simulink model "NDT_Localization"  (R2022a)
settings: Solver=FixedStepAuto  StartTime=0.0  StopTime=10.0  RelTol=1e-3
model workspace (MAT data in the model file):
  SL_ROS_VariableLengthArrays_MaxSizes : object (value not decoded)
undefined symbols (not defined in the file or in its folder): null
libraries: ros2lib x9, robotlib x8, simulink x1
(part 10 of 12)

== system NDT_Localization/observation_callback/check_localizer/If Action Subsystem/register_measurement_impl/If Action Subsystem/If Action Subsystem/solve/If Action Subsystem1/For Iterator Subsystem/compute_next_step/If Action Subsystem1/For Iterator Subsystem/If Action Subsystem/If Action Subsystem3/If Action Subsystem/f_u/For Iterator Subsystem/score ==
  score : Inport
  sigma : Inport  Port=2
  myu : Inport  Port=3
  x : Inport  Port=4
  d1 : Inport  Port=5
  d2 : Inport  Port=6
  Add : Sum  Inputs=+-
  Add1 : Sum
  Constant : Constant  Value=-2
  Divide1 : Product  Inputs=*/
  Gain : Gain  Gain=-1
  Math Function : Math
  Math Function1 : Math  Operator=transpose
  Math Function2 : Math  Operator=reciprocal
  Product : Product
  Product1 : Product  Inputs=3  Multiplication=Matrix(*)
  Product2 : Product
  p : Outport
  wires:
  sigma/1 -> Math Function2/1
  Math Function/1 -> Product/2
  Gain/1 -> Product/1  "-d1"
  myu/1 -> Add/2
  x/1 -> Add/1
  Product2/1 -> Math Function/1
  Add/1 -> Product1/3, Math Function1/1  "x-myu"
  Product/1 -> Add1/2
  Math Function1/1 -> Product1/1
  Product1/1 -> Product2/2
  Math Function2/1 -> Product1/2
  Constant/1 -> Divide1/2
  Divide1/1 -> Product2/1
  d2/1 -> Divide1/1  "d2"
  d1/1 -> Gain/1
  Add1/1 -> p/1
  score/1 -> Add1/1

== system NDT_Localization/observation_callback/check_localizer/If Action Subsystem/register_measurement_impl/If Action Subsystem/If Action Subsystem/solve/If Action Subsystem1/For Iterator Subsystem/compute_next_step/If Action Subsystem1/For Iterator Subsystem/If Action Subsystem/If Action Subsystem3/If Action Subsystem/f_u/angle_params/If Action Subsystem ==
  Action Port : ActionPort
  Constant : Constant
  Constant1 : Constant  Value=0
  Out1 : Outport
  Out2 : Outport  Port=2
  wires:
  Constant/1 -> Out1/1
  Constant1/1 -> Out2/1

== system NDT_Localization/observation_callback/check_localizer/If Action Subsystem/register_measurement_impl/If Action Subsystem/If Action Subsystem/solve/If Action Subsystem1/For Iterator Subsystem/compute_next_step/If Action Subsystem1/For Iterator Subsystem/If Action Subsystem/If Action Subsystem3/If Action Subsystem/f_u/angle_params/If Action Subsystem1 ==
  x : Inport
  Action Port : ActionPort
  Trigonometric Function : Trigonometry  Operator=cos
  Trigonometric Function1 : Trigonometry
  Out1 : Outport
  Out2 : Outport  Port=2
  wires:
  x/1 -> Trigonometric Function1/1, Trigonometric Function/1
  Trigonometric Function1/1 -> Out2/1
  Trigonometric Function/1 -> Out1/1

== system NDT_Localization/observation_callback/check_localizer/If Action Subsystem/register_measurement_impl/If Action Subsystem/If Action Subsystem/solve/If Action Subsystem1/For Iterator Subsystem/compute_next_step/If Action Subsystem1/For Iterator Subsystem/If Action Subsystem/If Action Subsystem3/If Action Subsystem/f_u/angle_params/If Action Subsystem2 ==
  Action Port : ActionPort
  Constant : Constant
  Constant1 : Constant  Value=0
  Out1 : Outport
  Out2 : Outport  Port=2
  wires:
  Constant/1 -> Out1/1
  Constant1/1 -> Out2/1

== system NDT_Localization/observation_callback/check_localizer/If Action Subsystem/register_measurement_impl/If Action Subsystem/If Action Subsystem/solve/If Action Subsystem1/For Iterator Subsystem/compute_next_step/If Action Subsystem1/For Iterator Subsystem/If Action Subsystem/If Action Subsystem3/If Action Subsystem/f_u/angle_params/If Action Subsystem3 ==
  y : Inport
  Action Port : ActionPort
  Trigonometric Function : Trigonometry  Operator=cos
  Trigonometric Function1 : Trigonometry
  Out1 : Outport
  Out2 : Outport  Port=2
  wires:
  Trigonometric Function/1 -> Out1/1
  Trigonometric Function1/1 -> Out2/1
  y/1 -> Trigonometric Function1/1, Trigonometric Function/1

== system NDT_Localization/observation_callback/check_localizer/If Action Subsystem/register_measurement_impl/If Action Subsystem/If Action Subsystem/solve/If Action Subsystem1/For Iterator Subsystem/compute_next_step/If Action Subsystem1/For Iterator Subsystem/If Action Subsystem/If Action Subsystem3/If Action Subsystem/f_u/angle_params/If Action Subsystem4 ==
  Action Port : ActionPort
  Constant : Constant
  Constant1 : Constant  Value=0
  Out1 : Outport
  Out2 : Outport  Port=2
  wires:
  Constant/1 -> Out1/1
  Constant1/1 -> Out2/1

== system NDT_Localization/observation_callback/check_localizer/If Action Subsystem/register_measurement_impl/If Action Subsystem/If Action Subsystem/solve/If Action Subsystem1/For Iterator Subsystem/compute_next_step/If Action Subsystem1/For Iterator Subsystem/If Action Subsystem/If Action Subsystem3/If Action Subsystem/f_u/angle_params/If Action Subsystem5 ==
  z : Inport
  Action Port : ActionPort
  Trigonometric Function : Trigonometry  Operator=cos
  Trigonometric Function1 : Trigonometry
  Out1 : Outport
  Out2 : Outport  Port=2
  wires:
  Trigonometric Function1/1 -> Out2/1
  Trigonometric Function/1 -> Out1/1
  z/1 -> Trigonometric Function1/1, Trigonometric Function/1

== system NDT_Localization/observation_callback/check_localizer/If Action Subsystem/register_measurement_impl/If Action Subsystem/If Action Subsystem/solve/If Action Subsystem1/For Iterator Subsystem/compute_next_step/If Action Subsystem1/For Iterator Subsystem/If Action Subsystem/If Action Subsystem3/psi_t/initial_objective_function/For Iterator Subsystem/gradient_jaco ==
  set_jacobian : Inport
  set_gradient : Inport  Port=2
  index : Inport  Port=3
  data : Inport  Port=4
  sigma : Inport  Port=5
  myu : Inport  Port=6
  x : Inport  Port=7
  d1 : Inport  Port=8
  d2 : Inport  Port=9
  Add : Sum  Inputs=+-
  Constant : Constant  Value=-2
  Divide1 : Product  Inputs=*/
  Math Function : Math
  Math Function1 : Math  Operator=transpose
  Math Function2 : Math  Operator=reciprocal
  Product : Product  Inputs=4
  Product1 : Product  Inputs=3  Multiplication=Matrix(*)
  Product2 : Product
  Product3 : Product
  Product4 : Product  Multiplication=Matrix(*)
  gradient_col : MATLAB Function  TreatAsAtomicUnit=on
  jaco_add : MATLAB Function  TreatAsAtomicUnit=on
  Out1 : Outport
  wires:
  myu/1 -> Add/2
  Constant/1 -> Divide1/2
  Math Function1/1 -> Product1/1
  Divide1/1 -> Product2/1
  d2/1 -> Divide1/1, Product/3  "d2"
  Math Function2/1 -> Product3/2, Product1/2  "inv_cov"
  Product1/1 -> Product2/2
  d1/1 -> Product/2  "d1"
  x/1 -> Add/1
  Math Function/1 -> Product/4
  Product2/1 -> Math Function/1
  Add/1 -> Product1/3, Math Function1/1  "x-myu"
  sigma/1 -> Math Function2/1
  Product/1 -> jaco_add/3(num)
  index/1 -> jaco_add/2(index), gradient_col/1(index)
  jaco_add/1(jacobian) -> Out1/1
  set_jacobian/1 -> jaco_add/1("jacobian ")
  set_gradient/1 -> gradient_col/2(gradient)
  gradient_col/1(y) -> Product3/1
  data/1 -> Product4/1
  Product3/1 -> Product4/2
  Product4/1 -> Product/1

== system NDT_Localization/observation_callback/check_localizer/If Action Subsystem/register_measurement_impl/If Action Subsystem/If Action Subsystem/solve/If Action Subsystem1/For Iterator Subsystem/compute_next_step/If Action Subsystem1/For Iterator Subsystem/If Action Subsystem/If Action Subsystem3/psi_t/initial_objective_function/For Iterator Subsystem/make_c_param ==
  outlier_ratio : Inport
  voxel_size_x : Inport  Port=2
  voxel_size_y : Inport  Port=3
  voxel_size_z : Inport  Port=4
  Constant : Constant
  Divide : Product  Inputs=*/
  Gain : Gain  Gain=10
  Product : Product  Inputs=3
  Subtract : Sum  Inputs=+-
  c1 : Outport
  c2 : Outport  Port=2
  wires:
  Constant/1 -> Subtract/1
  outlier_ratio/1 -> Divide/1, Subtract/2
  Subtract/1 -> Gain/1
  Gain/1 -> c1/1
  Product/1 -> Divide/2
  Divide/1 -> c2/1
  voxel_size_y/1 -> Product/2
  voxel_size_z/1 -> Product/3
  voxel_size_x/1 -> Product/1

== system NDT_Localization/observation_callback/check_localizer/If Action Subsystem/register_measurement_impl/If Action Subsystem/If Action Subsystem/solve/If Action Subsystem1/For Iterator Subsystem/compute_next_step/If Action Subsystem1/For Iterator Subsystem/If Action Subsystem/If Action Subsystem3/psi_t/initial_objective_function/For Iterator Subsystem/make_d_param ==
  c1 : Inport
  c2 : Inport  Port=2
  Add1 : Sum
  Add2 : Sum  Inputs=-+
  Add3 : Sum
  Add4 : Sum  Inputs=+-
  Constant : Constant  Value=-2
  Constant1 : Constant  Value=-0.5
  Divide : Product  Inputs=*/
  Math Function{3..4,6..7} (4 alike) : Math  Operator=log
  Math Function5 : Math
  Product3 : Product
  Product4 : Product
  d1 : Outport
  d2 : Outport  Port=2
  wires:
  Add2/1 -> Divide/2, d1/1  "d1"
  Math Function4/1 -> Add4/1, Add2/2  "-d3"
  Product4/1 -> Add3/1
  Add3/1 -> Math Function6/1
  c1/1 -> Product4/1, Add1/1
  Constant/1 -> Product3/2
  Constant1/1 -> Math Function5/1
  Product3/1 -> d2/1  "d2"
  Math Function5/1 -> Product4/2
  Math Function7/1 -> Product3/1
  Divide/1 -> Math Function7/1
  Math Function6/1 -> Add4/2
  c2/1 -> Add3/2, Math Function4/1, Add1/2
  Add4/1 -> Divide/1
  Add1/1 -> Math Function3/1
  Math Function3/1 -> Add2/1

== system NDT_Localization/observation_callback/check_localizer/If Action Subsystem/register_measurement_impl/If Action Subsystem/If Action Subsystem/solve/If Action Subsystem1/For Iterator Subsystem/compute_next_step/If Action Subsystem1/For Iterator Subsystem/If Action Subsystem/If Action Subsystem3/psi_t/initial_objective_function/For Iterator Subsystem/score ==
  score : Inport
  sigma : Inport  Port=2
  myu : Inport  Port=3
  x : Inport  Port=4
  d1 : Inport  Port=5
  d2 : Inport  Port=6
  Add : Sum  Inputs=+-
  Add1 : Sum
  Constant : Constant  Value=-2
  Divide1 : Product  Inputs=*/
  Gain : Gain  Gain=-1
  Math Function : Math
  Math Function1 : Math  Operator=transpose
  Math Function2 : Math  Operator=reciprocal
  Product : Product
  Product1 : Product  Inputs=3  Multiplication=Matrix(*)
  Product2 : Product
  p : Outport
  wires:
  sigma/1 -> Math Function2/1
  Math Function/1 -> Product/2
  Gain/1 -> Product/1  "-d1"
  myu/1 -> Add/2
  x/1 -> Add/1
  Product2/1 -> Math Function/1
  Add/1 -> Product1/3, Math Function1/1  "x-myu"
  Product/1 -> Add1/2
  Math Function1/1 -> Product1/1
  Product1/1 -> Product2/2
  Math Function2/1 -> Product1/2
  Constant/1 -> Divide1/2
  Divide1/1 -> Product2/1
  d2/1 -> Divide1/1  "d2"
  d1/1 -> Gain/1
  Add1/1 -> p/1
  score/1 -> Add1/1

== system NDT_Localization/observation_callback/check_localizer/If Action Subsystem/register_measurement_impl/If Action Subsystem/If Action Subsystem/solve/If Action Subsystem1/For Iterator Subsystem/compute_next_step/If Action Subsystem1/For Iterator Subsystem/If Action Subsystem/If Action Subsystem3/psi_t/initial_objective_function/angle_params/If Action Subsystem ==
  Action Port : ActionPort
  Constant : Constant
  Constant1 : Constant  Value=0
  Out1 : Outport
  Out2 : Outport  Port=2
  wires:
  Constant/1 -> Out1/1
  Constant1/1 -> Out2/1

== system NDT_Localization/observation_callback/check_localizer/If Action Subsystem/register_measurement_impl/If Action Subsystem/If Action Subsystem/solve/If Action Subsystem1/For Iterator Subsystem/compute_next_step/If Action Subsystem1/For Iterator Subsystem/If Action Subsystem/If Action Subsystem3/psi_t/initial_objective_function/angle_params/If Action Subsystem1 ==
  x : Inport
  Action Port : ActionPort
  Trigonometric Function : Trigonometry  Operator=cos
  Trigonometric Function1 : Trigonometry
  Out1 : Outport
  Out2 : Outport  Port=2
  wires:
  x/1 -> Trigonometric Function1/1, Trigonometric Function/1
  Trigonometric Function1/1 -> Out2/1
  Trigonometric Function/1 -> Out1/1

== system NDT_Localization/observation_callback/check_localizer/If Action Subsystem/register_measurement_impl/If Action Subsystem/If Action Subsystem/solve/If Action Subsystem1/For Iterator Subsystem/compute_next_step/If Action Subsystem1/For Iterator Subsystem/If Action Subsystem/If Action Subsystem3/psi_t/initial_objective_function/angle_params/If Action Subsystem2 ==
  Action Port : ActionPort
  Constant : Constant
  Constant1 : Constant  Value=0
  Out1 : Outport
  Out2 : Outport  Port=2
  wires:
  Constant/1 -> Out1/1
  Constant1/1 -> Out2/1

== system NDT_Localization/observation_callback/check_localizer/If Action Subsystem/register_measurement_impl/If Action Subsystem/If Action Subsystem/solve/If Action Subsystem1/For Iterator Subsystem/compute_next_step/If Action Subsystem1/For Iterator Subsystem/If Action Subsystem/If Action Subsystem3/psi_t/initial_objective_function/angle_params/If Action Subsystem3 ==
  y : Inport
  Action Port : ActionPort
  Trigonometric Function : Trigonometry  Operator=cos
  Trigonometric Function1 : Trigonometry
  Out1 : Outport
  Out2 : Outport  Port=2
  wires:
  Trigonometric Function/1 -> Out1/1
  Trigonometric Function1/1 -> Out2/1
  y/1 -> Trigonometric Function1/1, Trigonometric Function/1

== system NDT_Localization/observation_callback/check_localizer/If Action Subsystem/register_measurement_impl/If Action Subsystem/If Action Subsystem/solve/If Action Subsystem1/For Iterator Subsystem/compute_next_step/If Action Subsystem1/For Iterator Subsystem/If Action Subsystem/If Action Subsystem3/psi_t/initial_objective_function/angle_params/If Action Subsystem4 ==
  Action Port : ActionPort
  Constant : Constant
  Constant1 : Constant  Value=0
  Out1 : Outport
  Out2 : Outport  Port=2
  wires:
  Constant/1 -> Out1/1
  Constant1/1 -> Out2/1

== system NDT_Localization/observation_callback/check_localizer/If Action Subsystem/register_measurement_impl/If Action Subsystem/If Action Subsystem/solve/If Action Subsystem1/For Iterator Subsystem/compute_next_step/If Action Subsystem1/For Iterator Subsystem/If Action Subsystem/If Action Subsystem3/psi_t/initial_objective_function/angle_params/If Action Subsystem5 ==
  z : Inport
  Action Port : ActionPort
  Trigonometric Function : Trigonometry  Operator=cos
  Trigonometric Function1 : Trigonometry
  Out1 : Outport
  Out2 : Outport  Port=2
  wires:
  Trigonometric Function1/1 -> Out2/1
  Trigonometric Function/1 -> Out1/1
  z/1 -> Trigonometric Function1/1, Trigonometric Function/1

== system NDT_Localization/observation_callback/check_localizer/If Action Subsystem/register_measurement_impl/If Action Subsystem/If Action Subsystem/solve/If Action Subsystem1/For Iterator Subsystem/compute_next_step/If Action Subsystem1/For Iterator Subsystem/If Action Subsystem/If Action Subsystem3/psi_t/objective_function/For Iterator Subsystem/gradient_jaco ==
  set_jacobian : Inport
  set_gradient : Inport  Port=2
  index : Inport  Port=3
  data : Inport  Port=4
  sigma : Inport  Port=5
  myu : Inport  Port=6
  x : Inport  Port=7
  d1 : Inport  Port=8
  d2 : Inport  Port=9
  Add : Sum  Inputs=+-
  Constant : Constant  Value=-2
  Divide1 : Product  Inputs=*/
  Math Function : Math
  Math Function1 : Math  Operator=transpose
  Math Function2 : Math  Operator=reciprocal
  Product : Product  Inputs=4
  Product1 : Product  Inputs=3  Multiplication=Matrix(*)
  Product2 : Product
  Product3 : Product
  Product4 : Product  Multiplication=Matrix(*)
  gradient_col : MATLAB Function  TreatAsAtomicUnit=on
  jaco_add : MATLAB Function  TreatAsAtomicUnit=on
  Out1 : Outport
  wires:
  myu/1 -> Add/2
  Constant/1 -> Divide1/2
  Math Function1/1 -> Product1/1
  Divide1/1 -> Product2/1
  d2/1 -> Divide1/1, Product/3  "d2"
  Math Function2/1 -> Product3/2, Product1/2  "inv_cov"
  Product1/1 -> Product2/2
  d1/1 -> Product/2  "d1"
  x/1 -> Add/1
  Math Function/1 -> Product/4
  Product2/1 -> Math Function/1
  Add/1 -> Product1/3, Math Function1/1  "x-myu"
  sigma/1 -> Math Function2/1
  Product/1 -> jaco_add/3(num)
  index/1 -> jaco_add/2(index), gradient_col/1(index)
  jaco_add/1(jacobian) -> Out1/1
  set_jacobian/1 -> jaco_add/1("jacobian ")
  set_gradient/1 -> gradient_col/2(gradient)
  gradient_col/1(y) -> Product3/1
  data/1 -> Product4/1
  Product3/1 -> Product4/2
  Product4/1 -> Product/1

== system NDT_Localization/observation_callback/check_localizer/If Action Subsystem/register_measurement_impl/If Action Subsystem/If Action Subsystem/solve/If Action Subsystem1/For Iterator Subsystem/compute_next_step/If Action Subsystem1/For Iterator Subsystem/If Action Subsystem/If Action Subsystem3/psi_t/objective_function/For Iterator Subsystem/make_c_param ==
  outlier_ratio : Inport
  voxel_size_x : Inport  Port=2
  voxel_size_y : Inport  Port=3
  voxel_size_z : Inport  Port=4
  Constant : Constant
  Divide : Product  Inputs=*/
  Gain : Gain  Gain=10
  Product : Product  Inputs=3
  Subtract : Sum  Inputs=+-
  c1 : Outport
  c2 : Outport  Port=2
  wires:
  Constant/1 -> Subtract/1
  outlier_ratio/1 -> Divide/1, Subtract/2
  Subtract/1 -> Gain/1
  Gain/1 -> c1/1
  Product/1 -> Divide/2
  Divide/1 -> c2/1
  voxel_size_y/1 -> Product/2
  voxel_size_z/1 -> Product/3
  voxel_size_x/1 -> Product/1

== system NDT_Localization/observation_callback/check_localizer/If Action Subsystem/register_measurement_impl/If Action Subsystem/If Action Subsystem/solve/If Action Subsystem1/For Iterator Subsystem/compute_next_step/If Action Subsystem1/For Iterator Subsystem/If Action Subsystem/If Action Subsystem3/psi_t/objective_function/For Iterator Subsystem/make_d_param ==
  c1 : Inport
  c2 : Inport  Port=2
  Add1 : Sum
  Add2 : Sum  Inputs=-+
  Add3 : Sum
  Add4 : Sum  Inputs=+-
  Constant : Constant  Value=-2
  Constant1 : Constant  Value=-0.5
  Divide : Product  Inputs=*/
  Math Function{3..4,6..7} (4 alike) : Math  Operator=log
  Math Function5 : Math
  Product3 : Product
  Product4 : Product
  d1 : Outport
  d2 : Outport  Port=2
  wires:
  Add2/1 -> Divide/2, d1/1  "d1"
  Math Function4/1 -> Add4/1, Add2/2  "-d3"
  Product4/1 -> Add3/1
  Add3/1 -> Math Function6/1
  c1/1 -> Product4/1, Add1/1
  Constant/1 -> Product3/2
  Constant1/1 -> Math Function5/1
  Product3/1 -> d2/1  "d2"
  Math Function5/1 -> Product4/2
  Math Function7/1 -> Product3/1
  Divide/1 -> Math Function7/1
  Math Function6/1 -> Add4/2
  c2/1 -> Add3/2, Math Function4/1, Add1/2
  Add4/1 -> Divide/1
  Add1/1 -> Math Function3/1
  Math Function3/1 -> Add2/1

== system NDT_Localization/observation_callback/check_localizer/If Action Subsystem/register_measurement_impl/If Action Subsystem/If Action Subsystem/solve/If Action Subsystem1/For Iterator Subsystem/compute_next_step/If Action Subsystem1/For Iterator Subsystem/If Action Subsystem/If Action Subsystem3/psi_t/objective_function/For Iterator Subsystem/score ==
  score : Inport
  sigma : Inport  Port=2
  myu : Inport  Port=3
  x : Inport  Port=4
  d1 : Inport  Port=5
  d2 : Inport  Port=6
  Add : Sum  Inputs=+-
  Add1 : Sum
  Constant : Constant  Value=-2
  Divide1 : Product  Inputs=*/
  Gain : Gain  Gain=-1
  Math Function : Math
  Math Function1 : Math  Operator=transpose
  Math Function2 : Math  Operator=reciprocal
  Product : Product
  Product1 : Product  Inputs=3  Multiplication=Matrix(*)
  Product2 : Product
  p : Outport
  wires:
  sigma/1 -> Math Function2/1
  Math Function/1 -> Product/2
  Gain/1 -> Product/1  "-d1"
  myu/1 -> Add/2
  x/1 -> Add/1
  Product2/1 -> Math Function/1
  Add/1 -> Product1/3, Math Function1/1  "x-myu"
  Product/1 -> Add1/2
  Math Function1/1 -> Product1/1
  Product1/1 -> Product2/2
  Math Function2/1 -> Product1/2
  Constant/1 -> Divide1/2
  Divide1/1 -> Product2/1
  d2/1 -> Divide1/1  "d2"
  d1/1 -> Gain/1
  Add1/1 -> p/1
  score/1 -> Add1/1

== system NDT_Localization/observation_callback/check_localizer/If Action Subsystem/register_measurement_impl/If Action Subsystem/If Action Subsystem/solve/If Action Subsystem1/For Iterator Subsystem/compute_next_step/If Action Subsystem1/For Iterator Subsystem/If Action Subsystem/If Action Subsystem3/psi_t/objective_function/angle_params/If Action Subsystem ==
  Action Port : ActionPort
  Constant : Constant
  Constant1 : Constant  Value=0
  Out1 : Outport
  Out2 : Outport  Port=2
  wires:
  Constant/1 -> Out1/1
  Constant1/1 -> Out2/1

== system NDT_Localization/observation_callback/check_localizer/If Action Subsystem/register_measurement_impl/If Action Subsystem/If Action Subsystem/solve/If Action Subsystem1/For Iterator Subsystem/compute_next_step/If Action Subsystem1/For Iterator Subsystem/If Action Subsystem/If Action Subsystem3/psi_t/objective_function/angle_params/If Action Subsystem1 ==
  x : Inport
  Action Port : ActionPort
  Trigonometric Function : Trigonometry  Operator=cos
  Trigonometric Function1 : Trigonometry
  Out1 : Outport
  Out2 : Outport  Port=2
  wires:
  x/1 -> Trigonometric Function1/1, Trigonometric Function/1
  Trigonometric Function1/1 -> Out2/1
  Trigonometric Function/1 -> Out1/1

== system NDT_Localization/observation_callback/check_localizer/If Action Subsystem/register_measurement_impl/If Action Subsystem/If Action Subsystem/solve/If Action Subsystem1/For Iterator Subsystem/compute_next_step/If Action Subsystem1/For Iterator Subsystem/If Action Subsystem/If Action Subsystem3/psi_t/objective_function/angle_params/If Action Subsystem2 ==
  Action Port : ActionPort
  Constant : Constant
  Constant1 : Constant  Value=0
  Out1 : Outport
  Out2 : Outport  Port=2
  wires:
  Constant/1 -> Out1/1
  Constant1/1 -> Out2/1

== system NDT_Localization/observation_callback/check_localizer/If Action Subsystem/register_measurement_impl/If Action Subsystem/If Action Subsystem/solve/If Action Subsystem1/For Iterator Subsystem/compute_next_step/If Action Subsystem1/For Iterator Subsystem/If Action Subsystem/If Action Subsystem3/psi_t/objective_function/angle_params/If Action Subsystem3 ==
  y : Inport
  Action Port : ActionPort
  Trigonometric Function : Trigonometry  Operator=cos
  Trigonometric Function1 : Trigonometry
  Out1 : Outport
  Out2 : Outport  Port=2
  wires:
  Trigonometric Function/1 -> Out1/1
  Trigonometric Function1/1 -> Out2/1
  y/1 -> Trigonometric Function1/1, Trigonometric Function/1

== system NDT_Localization/observation_callback/check_localizer/If Action Subsystem/register_measurement_impl/If Action Subsystem/If Action Subsystem/solve/If Action Subsystem1/For Iterator Subsystem/compute_next_step/If Action Subsystem1/For Iterator Subsystem/If Action Subsystem/If Action Subsystem3/psi_t/objective_function/angle_params/If Action Subsystem4 ==
  Action Port : ActionPort
  Constant : Constant
  Constant1 : Constant  Value=0
  Out1 : Outport
  Out2 : Outport  Port=2
  wires:
  Constant/1 -> Out1/1
  Constant1/1 -> Out2/1

== system NDT_Localization/observation_callback/check_localizer/If Action Subsystem/register_measurement_impl/If Action Subsystem/If Action Subsystem/solve/If Action Subsystem1/For Iterator Subsystem/compute_next_step/If Action Subsystem1/For Iterator Subsystem/If Action Subsystem/If Action Subsystem3/psi_t/objective_function/angle_params/If Action Subsystem5 ==
  z : Inport
  Action Port : ActionPort
  Trigonometric Function : Trigonometry  Operator=cos
  Trigonometric Function1 : Trigonometry
  Out1 : Outport
  Out2 : Outport  Port=2
  wires:
  Trigonometric Function1/1 -> Out2/1
  Trigonometric Function/1 -> Out1/1
  z/1 -> Trigonometric Function1/1, Trigonometric Function/1

== matlab function NDT_Localization/observation_callback/check_localizer/If Action Subsystem/register_measurement_impl/If Action Subsystem/If Action Subsystem/solve/If Action Subsystem1/For Iterator Subsystem/compute_next_step/If Action Subsystem1/For Iterator Subsystem/If Action Subsystem/If Action Subsystem3/psi_t/initial_objective_function/For Iterator Subsystem/gradient_jaco/gradient_col ==
  data: index input; gradient input; y output
function y = fcn(index,gradient)

y = gradient(:,index);

== matlab function NDT_Localization/observation_callback/check_localizer/If Action Subsystem/register_measurement_impl/If Action Subsystem/If Action Subsystem/solve/If Action Subsystem1/For Iterator Subsystem/compute_next_step/If Action Subsystem1/For Iterator Subsystem/If Action Subsystem/If Action Subsystem3/psi_t/initial_objective_function/For Iterator Subsystem/gradient_jaco/jaco_add ==
  data: jacobian input; jacobian output; index input; num input
function jacobian = fcn(jacobian,index,num)

jacobian(index) = jacobian(index)+num;

== matlab function NDT_Localization/observation_callback/check_localizer/If Action Subsystem/register_measurement_impl/If Action Subsystem/If Action Subsystem/insert/If Action Subsystem/MATLAB Function ==
  data: msg input; points output
function points= fcn(msg)

points = reshape(msg,1,size(msg));

== matlab function NDT_Localization/observation_callback/check_localizer/If Action Subsystem/register_measurement_impl/If Action Subsystem/If Action Subsystem/solve/If Action Subsystem1/For Iterator Subsystem/compute_next_step/If Action Subsystem1/For Iterator Subsystem/If Action Subsystem/If Action Subsystem3/psi_t/initial_objective_function/angle_params/MATLAB Function ==
  data: x output; u input; y output; z output
function [x,y,z] = fcn(u)
x = u(3);
y = u(4);
z = u(5);

== matlab function NDT_Localization/observation_callback/check_localizer/If Action Subsystem/register_measurement_impl/If Action Subsystem/If Action Subsystem/solve/If Action Subsystem1/For Iterator Subsystem/compute_next_step/If Action Subsystem1/For Iterator Subsystem/If Action Subsystem/If Action Subsystem3/psi_t/initial_objective_function/gradient_angle/ga_a ==
  data: x input; out output; y input; z input
function out = fcn(x, y, z)
out = zeros(1,3); 
out(1) = x;
out(2) = y;
out(3) = z;

== matlab function NDT_Localization/observation_callback/check_localizer/If Action Subsystem/register_measurement_impl/If Action Subsystem/If Action Subsystem/solve/If Action Subsystem1/For Iterator Subsystem/compute_next_step/If Action Subsystem1/For Iterator Subsystem/If Action Subsystem/If Action Subsystem3/psi_t/initial_objective_function/gradient_angle/ga_b ==
  data: x input; out output; y input; z input
function out = fcn(x, y, z)
out = zeros(1,3); 
out(1) = x;
out(2) = y;
out(3) = z;

== matlab function NDT_Localization/observation_callback/check_localizer/If Action Subsystem/register_measurement_impl/If Action Subsystem/If Action Subsystem/solve/If Action Subsystem1/For Iterator Subsystem/compute_next_step/If Action Subsystem1/For Iterator Subsystem/If Action Subsystem/If Action Subsystem3/psi_t/initial_objective_function/gradient_angle/ga_c ==
  data: x input; out output; y input; z input
function out = fcn(x, y, z)
out = zeros(1,3); 
out(1) = x;
out(2) = y;
out(3) = z;

== matlab function NDT_Localization/observation_callback/check_localizer/If Action Subsystem/register_measurement_impl/If Action Subsystem/If Action Subsystem/solve/If Action Subsystem1/For Iterator Subsystem/compute_next_step/If Action Subsystem1/For Iterator Subsystem/If Action Subsystem/If Action Subsystem3/psi_t/initial_objective_function/gradient_angle/ga_d ==
  data: x input; out output; y input; z input
function out = fcn(x, y, z)
out = zeros(1,3); 
out(1) = x;
out(2) = y;
out(3) = z;

== matlab function NDT_Localization/observation_callback/check_localizer/If Action Subsystem/register_measurement_impl/If Action Subsystem/If Action Subsystem/solve/If Action Subsystem1/For Iterator Subsystem/compute_next_step/If Action Subsystem1/For Iterator Subsystem/If Action Subsystem/If Action Subsystem3/psi_t/initial_objective_function/gradient_angle/ga_e ==
  data: x input; out output; y input; z input
function out = fcn(x, y, z)
out = zeros(1,3); 
out(1) = x;
out(2) = y;
out(3) = z;

== matlab function NDT_Localization/observation_callback/check_localizer/If Action Subsystem/register_measurement_impl/If Action Subsystem/If Action Subsystem/solve/If Action Subsystem1/For Iterator Subsystem/compute_next_step/If Action Subsystem1/For Iterator Subsystem/If Action Subsystem/If Action Subsystem3/psi_t/initial_objective_function/gradient_angle/ga_f ==
  data: x input; out output; y input; z input
function out = fcn(x, y, z)
out = zeros(1,3); 
out(1) = x;
out(2) = y;
out(3) = z;

== matlab function NDT_Localization/observation_callback/check_localizer/If Action Subsystem/register_measurement_impl/If Action Subsystem/If Action Subsystem/solve/is_valid_probability/MATLAB Function ==
  data: u input; y output
function y = fcn(u)

y = isnan(u);

== matlab function NDT_Localization/observation_callback/check_localizer/If Action Subsystem/register_measurement_impl/If Action Subsystem/If Action Subsystem/solve/If Action Subsystem1/For Iterator Subsystem/compute_next_step/If Action Subsystem1/For Iterator Subsystem/If Action Subsystem/If Action Subsystem3/psi_t/initial_objective_function/gradient_angle/ga_g ==
  data: x input; out output; y input; z input
function out = fcn(x, y, z)
out = zeros(1,3); 
out(1) = x;
out(2) = y;
out(3) = z;

== matlab function NDT_Localization/observation_callback/check_localizer/If Action Subsystem/register_measurement_impl/If Action Subsystem/If Action Subsystem/solve/If Action Subsystem1/For Iterator Subsystem/compute_next_step/If Action Subsystem1/For Iterator Subsystem/If Action Subsystem/If Action Subsystem3/psi_t/initial_objective_function/gradient_angle/ga_h ==
  data: x input; out output; y input; z input
function out = fcn(x, y, z)
out = zeros(1,3); 
out(1) = x;
out(2) = y;
out(3) = z;

== matlab function NDT_Localization/observation_callback/check_localizer/If Action Subsystem/register_measurement_impl/If Action Subsystem/If Action Subsystem/solve/If Action Subsystem1/For Iterator Subsystem/compute_next_step/If Action Subsystem1/For Iterator Subsystem/If Action Subsystem/If Action Subsystem3/psi_t/initial_objective_function/point_gradient ==
  data: hessian output; ga_a input; ga_b input; ga_c input; ga_d input; ga_e input; ga_f input; ga_g input; ga_h input
function hessian = fcn(ga_a, ga_b, ga_c, ga_d, ga_e, ga_f, ga_g, ga_h)

hessian = zeros(3,6,"single");
hessian(1,3) = ga_a;
hessian(2,3) = ga_b;
hessian(0,4) = ga_c;
hessian(1,4) = ga_d;
hessian(2,4) = ga_e;
hessian(0,5) = ga_f;
hessian(1,5) = ga_g;
hessian(2,5) = ga_h;

== matlab function NDT_Localization/observation_callback/check_localizer/If Action Subsystem/register_measurement_impl/If Action Subsystem/If Action Subsystem/solve/If Action Subsystem1/For Iterator Subsystem/compute_next_step/If Action Subsystem1/For Iterator Subsystem/If Action Subsystem/If Action Subsystem3/psi_t/initial_objective_function/set_jacobian ==
  data: jacobian output
function jacobian = fcn()

jacobian = zeros(6,1,"single");

== matlab function NDT_Localization/observation_callback/check_localizer/If Action Subsystem/register_measurement_impl/If Action Subsystem/If Action Subsystem/solve/If Action Subsystem1/For Iterator Subsystem/compute_next_step/If Action Subsystem1/For Iterator Subsystem/If Action Subsystem/If Action Subsystem3/psi_t/objective_function/For Iterator Subsystem/Affine ==
  data: out output; u input
function out = fcn(u)

tform = affine3d;
pt = pointCloud(u);
xyz = pctransform(pt,tform);
out = xyz.Location;

== matlab function NDT_Localization/observation_callback/check_localizer/If Action Subsystem/register_measurement_impl/If Action Subsystem/If Action Subsystem/solve/If Action Subsystem1/For Iterator Subsystem/compute_next_step/If Action Subsystem1/For Iterator Subsystem/If Action Subsystem/If Action Subsystem3/psi_t/objective_function/For Iterator Subsystem/MATLAB Function ==
  data: data input; pt output; index input
function pt = fcn(data,index)

pt = data(index);

== matlab function NDT_Localization/observation_callback/check_localizer/If Action Subsystem/register_measurement_impl/If Action Subsystem/If Action Subsystem/solve/If Action Subsystem1/For Iterator Subsystem/compute_next_step/If Action Subsystem1/For Iterator Subsystem/If Action Subsystem/If Action Subsystem3/psi_t/objective_function/For Iterator Subsystem/gradient_jaco/gradient_col ==
  data: index input; gradient input; y output
function y = fcn(index,gradient)

y = gradient(:,index);

== matlab function NDT_Localization/observation_callback/check_localizer/If Action Subsystem/register_measurement_impl/If Action Subsystem/If Action Subsystem/solve/If Action Subsystem1/For Iterator Subsystem/compute_next_step/If Action Subsystem1/For Iterator Subsystem/If Action Subsystem/If Action Subsystem3/psi_t/objective_function/For Iterator Subsystem/gradient_jaco/jaco_add ==
  data: jacobian input; jacobian output; index input; num input
function jacobian = fcn(jacobian,index,num)

jacobian(index) = jacobian(index)+num;

== matlab function NDT_Localization/map_callback/check_localizer/set_map/set_map_impl/insert/insert_/If Action Subsystem/While Iterator Subsystem/index/MATLAB Function ==
  data: x output; u input; y output; z output
function [x,y,z] = fcn(u)

x = u(1);
y = u(2);
z = u(3);

== matlab function NDT_Localization/observation_callback/check_localizer/If Action Subsystem/register_measurement_impl/If Action Subsystem/If Action Subsystem/solve/If Action Subsystem1/For Iterator Subsystem/compute_next_step/If Action Subsystem1/For Iterator Subsystem/If Action Subsystem/If Action Subsystem3/psi_t/objective_function/angle_params/MATLAB Function ==
  data: x output; u input; y output; z output
function [x,y,z] = fcn(u)
x = u(3);
y = u(4);
z = u(5);

== matlab function NDT_Localization/observation_callback/check_localizer/If Action Subsystem/register_measurement_impl/If Action Subsystem/If Action Subsystem/solve/If Action Subsystem1/For Iterator Subsystem/compute_next_step/If Action Subsystem1/For Iterator Subsystem/If Action Subsystem/If Action Subsystem3/psi_t/objective_function/gradient_angle/ga_a ==
  data: x input; out output; y input; z input
function out = fcn(x, y, z)
out = zeros(1,3); 
out(1) = x;
out(2) = y;
out(3) = z;

== matlab function NDT_Localization/observation_callback/check_localizer/If Action Subsystem/register_measurement_impl/If Action Subsystem/If Action Subsystem/solve/If Action Subsystem1/For Iterator Subsystem/compute_next_step/If Action Subsystem1/For Iterator Subsystem/If Action Subsystem/If Action Subsystem3/psi_t/objective_function/gradient_angle/ga_b ==
  data: x input; out output; y input; z input
function out = fcn(x, y, z)
out = zeros(1,3); 
out(1) = x;
out(2) = y;
out(3) = z;

== matlab function NDT_Localization/observation_callback/check_localizer/If Action Subsystem/register_measurement_impl/If Action Subsystem/If Action Subsystem/solve/If Action Subsystem1/For Iterator Subsystem/compute_next_step/If Action Subsystem1/For Iterator Subsystem/If Action Subsystem/If Action Subsystem3/psi_t/objective_function/gradient_angle/ga_c ==
  data: x input; out output; y input; z input
function out = fcn(x, y, z)
out = zeros(1,3); 
out(1) = x;
out(2) = y;
out(3) = z;

== matlab function NDT_Localization/observation_callback/check_localizer/If Action Subsystem/register_measurement_impl/If Action Subsystem/If Action Subsystem/solve/If Action Subsystem1/For Iterator Subsystem/compute_next_step/If Action Subsystem1/For Iterator Subsystem/If Action Subsystem/If Action Subsystem3/psi_t/objective_function/gradient_angle/ga_d ==
  data: x input; out output; y input; z input
function out = fcn(x, y, z)
out = zeros(1,3); 
out(1) = x;
out(2) = y;
out(3) = z;

== matlab function NDT_Localization/observation_callback/check_localizer/If Action Subsystem/register_measurement_impl/If Action Subsystem/If Action Subsystem/solve/If Action Subsystem1/For Iterator Subsystem/compute_next_step/If Action Subsystem1/For Iterator Subsystem/If Action Subsystem/If Action Subsystem3/psi_t/objective_function/gradient_angle/ga_e ==
  data: x input; out output; y input; z input
function out = fcn(x, y, z)
out = zeros(1,3); 
out(1) = x;
out(2) = y;
out(3) = z;

== matlab function NDT_Localization/observation_callback/check_localizer/If Action Subsystem/register_measurement_impl/If Action Subsystem/If Action Subsystem/solve/If Action Subsystem1/For Iterator Subsystem/compute_next_step/If Action Subsystem1/For Iterator Subsystem/If Action Subsystem/If Action Subsystem3/psi_t/objective_function/gradient_angle/ga_f ==
  data: x input; out output; y input; z input
function out = fcn(x, y, z)
out = zeros(1,3); 
out(1) = x;
out(2) = y;
out(3) = z;

== matlab function NDT_Localization/observation_callback/check_localizer/If Action Subsystem/register_measurement_impl/If Action Subsystem/If Action Subsystem/solve/If Action Subsystem1/For Iterator Subsystem/compute_next_step/If Action Subsystem1/For Iterator Subsystem/If Action Subsystem/If Action Subsystem3/psi_t/objective_function/gradient_angle/ga_g ==
  data: x input; out output; y input; z input
function out = fcn(x, y, z)
out = zeros(1,3); 
out(1) = x;
out(2) = y;
out(3) = z;

== matlab function NDT_Localization/observation_callback/check_localizer/If Action Subsystem/register_measurement_impl/If Action Subsystem/If Action Subsystem/solve/If Action Subsystem1/For Iterator Subsystem/compute_next_step/If Action Subsystem1/For Iterator Subsystem/If Action Subsystem/If Action Subsystem3/psi_t/objective_function/gradient_angle/ga_h ==
  data: x input; out output; y input; z input
function out = fcn(x, y, z)
out = zeros(1,3); 
out(1) = x;
out(2) = y;
out(3) = z;

== matlab function NDT_Localization/observation_callback/check_localizer/If Action Subsystem/register_measurement_impl/If Action Subsystem/If Action Subsystem/solve/If Action Subsystem1/For Iterator Subsystem/compute_next_step/If Action Subsystem1/For Iterator Subsystem/If Action Subsystem/If Action Subsystem3/psi_t/objective_function/point_gradient ==
  data: hessian output; ga_a input; ga_b input; ga_c input; ga_d input; ga_e input; ga_f input; ga_g input; ga_h input
function hessian = fcn(ga_a, ga_b, ga_c, ga_d, ga_e, ga_f, ga_g, ga_h)

hessian = zeros(3,6,"single");
hessian(1,3) = ga_a;
hessian(2,3) = ga_b;
hessian(0,4) = ga_c;
hessian(1,4) = ga_d;
hessian(2,4) = ga_e;
hessian(0,5) = ga_f;
hessian(1,5) = ga_g;
hessian(2,5) = ga_h;

== matlab function NDT_Localization/map_callback/check_localizer/set_map/set_map_impl/insert/insert_/If Action Subsystem/While Iterator Subsystem/index/FEPS ==
  data: y output
function y = fcn()

y = eps();

== matlab function NDT_Localization/observation_callback/check_localizer/If Action Subsystem/register_measurement_impl/If Action Subsystem/If Action Subsystem/solve/If Action Subsystem1/For Iterator Subsystem/compute_next_step/If Action Subsystem1/For Iterator Subsystem/If Action Subsystem/If Action Subsystem3/psi_t/objective_function/set_jacobian ==
  data: jacobian output
function jacobian = fcn()

jacobian = zeros(6,1,"single");

== matlab function NDT_Localization/observation_callback/check_localizer/If Action Subsystem/register_measurement_impl/If Action Subsystem/If Action Subsystem/solve/If Action Subsystem1/For Iterator Subsystem/compute_next_step/If Action Subsystem1/For Iterator Subsystem/If Action Subsystem/If Action Subsystem3/If Action Subsystem/f_l/For Iterator Subsystem/Affine ==
  data: out output; u input
function out = fcn(u)

tform = affine3d;
pt = pointCloud(u);
xyz = pctransform(pt,tform);
out = xyz.Location;

== matlab function NDT_Localization/observation_callback/check_localizer/If Action Subsystem/register_measurement_impl/If Action Subsystem/If Action Subsystem/solve/If Action Subsystem1/For Iterator Subsystem/compute_next_step/If Action Subsystem1/For Iterator Subsystem/If Action Subsystem/If Action Subsystem3/If Action Subsystem/f_l/For Iterator Subsystem/MATLAB Function ==
  data: data input; pt output; index input
function pt = fcn(data,index)

pt = data(index);

== matlab function NDT_Localization/observation_callback/check_localizer/If Action Subsystem/register_measurement_impl/If Action Subsystem/If Action Subsystem/solve/If Action Subsystem1/For Iterator Subsystem/compute_next_step/If Action Subsystem1/For Iterator Subsystem/If Action Subsystem/If Action Subsystem3/If Action Subsystem/f_l/For Iterator Subsystem/gradient_jaco/gradient_col ==
  data: index input; gradient input; y output
function y = fcn(index,gradient)

y = gradient(:,index);

== matlab function NDT_Localization/observation_callback/check_localizer/If Action Subsystem/register_measurement_impl/If Action Subsystem/If Action Subsystem/solve/If Action Subsystem1/For Iterator Subsystem/compute_next_step/If Action Subsystem1/For Iterator Subsystem/If Action Subsystem/If Action Subsystem3/If Action Subsystem/f_l/For Iterator Subsystem/gradient_jaco/jaco_add ==
  data: jacobian input; jacobian output; index input; num input
function jacobian = fcn(jacobian,index,num)

jacobian(index) = jacobian(index)+num;

== matlab function NDT_Localization/observation_callback/check_localizer/If Action Subsystem/register_measurement_impl/If Action Subsystem/If Action Subsystem/solve/If Action Subsystem1/For Iterator Subsystem/compute_next_step/If Action Subsystem1/For Iterator Subsystem/If Action Subsystem/If Action Subsystem3/If Action Subsystem/f_l/angle_params/MATLAB Function ==
  data: x output; u input; y output; z output
function [x,y,z] = fcn(u)
x = u(3);
y = u(4);
z = u(5);

== matlab function NDT_Localization/observation_callback/check_localizer/If Action Subsystem/register_measurement_impl/If Action Subsystem/If Action Subsystem/solve/If Action Subsystem1/For Iterator Subsystem/compute_next_step/If Action Subsystem1/For Iterator Subsystem/If Action Subsystem/If Action Subsystem3/If Action Subsystem/f_l/gradient_angle/ga_a ==
  data: x input; out output; y input; z input
function out = fcn(x, y, z)
out = zeros(1,3); 
out(1) = x;
out(2) = y;
out(3) = z;

== matlab function NDT_Localization/initial_pose_callback/lookupTransform/if_true/MATLAB Function ==
  data: now output
function now = ros2_time

rclcpp::Clock system_clock(rcl_clock_type_t RCL_SYSTEM_TIME);
rclcpp::Time now = system_clock.now();

end

== matlab function NDT_Localization/observation_callback/check_localizer/If Action Subsystem/register_measurement_impl/If Action Subsystem/If Action Subsystem/solve/If Action Subsystem1/For Iterator Subsystem/compute_next_step/If Action Subsystem1/For Iterator Subsystem/If Action Subsystem/If Action Subsystem3/If Action Subsystem/f_l/gradient_angle/ga_b ==
  data: x input; out output; y input; z input
function out = fcn(x, y, z)
out = zeros(1,3); 
out(1) = x;
out(2) = y;
out(3) = z;

== matlab function NDT_Localization/observation_callback/check_localizer/If Action Subsystem/register_measurement_impl/If Action Subsystem/If Action Subsystem/solve/If Action Subsystem1/For Iterator Subsystem/compute_next_step/If Action Subsystem1/For Iterator Subsystem/If Action Subsystem/If Action Subsystem3/If Action Subsystem/f_l/gradient_angle/ga_c ==
  data: x input; out output; y input; z input
function out = fcn(x, y, z)
out = zeros(1,3); 
out(1) = x;
out(2) = y;
out(3) = z;

== matlab function NDT_Localization/observation_callback/check_localizer/If Action Subsystem/register_measurement_impl/If Action Subsystem/If Action Subsystem/solve/If Action Subsystem1/For Iterator Subsystem/compute_next_step/If Action Subsystem1/For Iterator Subsystem/If Action Subsystem/If Action Subsystem3/If Action Subsystem/f_l/gradient_angle/ga_d ==
  data: x input; out output; y input; z input
function out = fcn(x, y, z)
out = zeros(1,3); 
out(1) = x;
out(2) = y;
out(3) = z;

== matlab function NDT_Localization/observation_callback/check_localizer/If Action Subsystem/register_measurement_impl/If Action Subsystem/If Action Subsystem/solve/If Action Subsystem1/For Iterator Subsystem/compute_next_step/If Action Subsystem1/For Iterator Subsystem/If Action Subsystem/If Action Subsystem3/If Action Subsystem/f_l/gradient_angle/ga_e ==
  data: x input; out output; y input; z input
function out = fcn(x, y, z)
out = zeros(1,3); 
out(1) = x;
out(2) = y;
out(3) = z;

== matlab function NDT_Localization/observation_callback/check_localizer/If Action Subsystem/register_measurement_impl/If Action Subsystem/If Action Subsystem/solve/If Action Subsystem1/For Iterator Subsystem/compute_next_step/If Action Subsystem1/For Iterator Subsystem/If Action Subsystem/If Action Subsystem3/If Action Subsystem/f_l/gradient_angle/ga_f ==
  data: x input; out output; y input; z input
function out = fcn(x, y, z)
out = zeros(1,3); 
out(1) = x;
out(2) = y;
out(3) = z;

== matlab function NDT_Localization/observation_callback/check_localizer/If Action Subsystem/register_measurement_impl/If Action Subsystem/If Action Subsystem/solve/If Action Subsystem1/For Iterator Subsystem/compute_next_step/If Action Subsystem1/For Iterator Subsystem/If Action Subsystem/If Action Subsystem3/If Action Subsystem/f_l/gradient_angle/ga_g ==
  data: x input; out output; y input; z input
function out = fcn(x, y, z)
out = zeros(1,3); 
out(1) = x;
out(2) = y;
out(3) = z;

== matlab function NDT_Localization/observation_callback/check_localizer/If Action Subsystem/register_measurement_impl/If Action Subsystem/If Action Subsystem/solve/If Action Subsystem1/For Iterator Subsystem/compute_next_step/If Action Subsystem1/For Iterator Subsystem/If Action Subsystem/If Action Subsystem3/If Action Subsystem/f_l/gradient_angle/ga_h ==
  data: x input; out output; y input; z input
function out = fcn(x, y, z)
out = zeros(1,3); 
out(1) = x;
out(2) = y;
out(3) = z;

== matlab function NDT_Localization/observation_callback/check_localizer/If Action Subsystem/register_measurement_impl/If Action Subsystem/If Action Subsystem/solve/set_hessian ==
  data: hessian output
function hessian = fcn()

hessian = zeros(6,6,"single");

== matlab function NDT_Localization/observation_callback/check_localizer/If Action Subsystem/register_measurement_impl/If Action Subsystem/If Action Subsystem/solve/If Action Subsystem1/For Iterator Subsystem/compute_next_step/If Action Subsystem1/For Iterator Subsystem/If Action Subsystem/If Action Subsystem3/If Action Subsystem/f_l/point_gradient ==
  data: hessian output; ga_a input; ga_b input; ga_c input; ga_d input; ga_e input; ga_f input; ga_g input; ga_h input
function hessian = fcn(ga_a, ga_b, ga_c, ga_d, ga_e, ga_f, ga_g, ga_h)

hessian = zeros(3,6,"single");
hessian(1,3) = ga_a;
hessian(2,3) = ga_b;
hessian(0,4) = ga_c;
hessian(1,4) = ga_d;
hessian(2,4) = ga_e;
hessian(0,5) = ga_f;
hessian(1,5) = ga_g;
hessian(2,5) = ga_h;

== matlab function NDT_Localization/observation_callback/check_localizer/If Action Subsystem/register_measurement_impl/If Action Subsystem/If Action Subsystem/solve/If Action Subsystem1/For Iterator Subsystem/compute_next_step/If Action Subsystem1/For Iterator Subsystem/If Action Subsystem/If Action Subsystem3/If Action Subsystem/f_l/set_jacobian ==
  data: jacobian output
function jacobian = fcn()

jacobian = zeros(6,1,"single");

== matlab function NDT_Localization/observation_callback/check_localizer/If Action Subsystem/register_measurement_impl/If Action Subsystem/If Action Subsystem/solve/If Action Subsystem1/For Iterator Subsystem/compute_next_step/If Action Subsystem1/For Iterator Subsystem/If Action Subsystem/If Action Subsystem3/If Action Subsystem/f_u/For Iterator Subsystem/Affine ==
  data: out output; u input
function out = fcn(u)

tform = affine3d;
pt = pointCloud(u);
xyz = pctransform(pt,tform);
out = xyz.Location;

== matlab function NDT_Localization/observation_callback/check_localizer/If Action Subsystem/register_measurement_impl/If Action Subsystem/If Action Subsystem/solve/If Action Subsystem1/For Iterator Subsystem/compute_next_step/If Action Subsystem1/For Iterator Subsystem/If Action Subsystem/If Action Subsystem3/If Action Subsystem/f_u/For Iterator Subsystem/MATLAB Function ==
  data: data input; pt output; index input
function pt = fcn(data,index)

pt = data(index);

== matlab function NDT_Localization/observation_callback/check_localizer/If Action Subsystem/register_measurement_impl/If Action Subsystem/If Action Subsystem/solve/If Action Subsystem1/For Iterator Subsystem/compute_next_step/If Action Subsystem1/For Iterator Subsystem/If Action Subsystem/If Action Subsystem3/If Action Subsystem/f_u/For Iterator Subsystem/gradient_jaco/gradient_col ==
  data: index input; gradient input; y output
function y = fcn(index,gradient)

y = gradient(:,index);

== matlab function NDT_Localization/observation_callback/check_localizer/If Action Subsystem/register_measurement_impl/If Action Subsystem/If Action Subsystem/solve/If Action Subsystem1/For Iterator Subsystem/compute_next_step/If Action Subsystem1/For Iterator Subsystem/If Action Subsystem/If Action Subsystem3/If Action Subsystem/f_u/For Iterator Subsystem/gradient_jaco/jaco_add ==
  data: jacobian input; jacobian output; index input; num input
function jacobian = fcn(jacobian,index,num)

jacobian(index) = jacobian(index)+num;

== matlab function NDT_Localization/observation_callback/check_localizer/If Action Subsystem/register_measurement_impl/If Action Subsystem/If Action Subsystem/solve/If Action Subsystem1/For Iterator Subsystem/compute_next_step/If Action Subsystem1/For Iterator Subsystem/If Action Subsystem/If Action Subsystem3/If Action Subsystem/f_u/angle_params/MATLAB Function ==
  data: x output; u input; y output; z output
function [x,y,z] = fcn(u)
x = u(3);
y = u(4);
z = u(5);

== matlab function NDT_Localization/observation_callback/check_localizer/If Action Subsystem/register_measurement_impl/If Action Subsystem/If Action Subsystem/solve/If Action Subsystem1/For Iterator Subsystem/For Iterator Subsystem/Affine ==
  data: out output; u input
function out = fcn(u)

tform = affine3d;
pt = pointCloud(u);
xyz = pctransform(pt,tform);
out = xyz.Location;
